simulink library "Mako_Lib"  (R2024b)
settings: Solver=VariableStepAuto  StartTime=0.0  StopTime=10.0  RelTol=1e-3
settings Model: Creator=pinto  LastModifiedBy=pinto

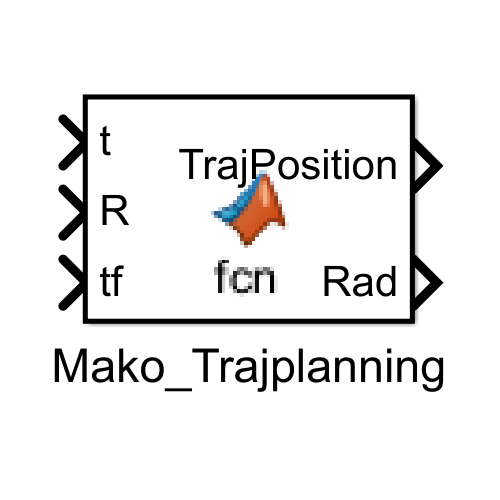
[thumbnail: Simulink's stored preview of the top-level diagram]
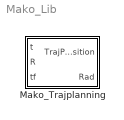
== system Mako_Lib ==
  Mako_Trajplanning : MATLAB Function  TreatAsAtomicUnit=on

== matlab function Mako_Lib/Mako_Trajplanning ==
  data: t input; TrajPosition output; R input; tf input; Rad output
function [TrajPosition,Rad] = Mako_Trajplanning(t,R,tf)
%#codegen

%    This function was generated by the Symbolic Math Toolbox version 24.2.
%    11-Jun-2025 20:14:08

% t = complex(t);  % if required to enforce complex operations
% R = complex(R);  % if required to enforce complex operations
% tf = complex(tf);  % if required to enforce complex operations
t2 = t.^2;
t3 = t.^3;
t4 = tf.^3;
t5 = 1.0./R;
t6 = 1.0./tf.^2;
t9 = sqrt(2.0);
t10 = pi.*(3.0./4.0);
t23 = R.*6.71238898038469;
t7 = 1.0./t4;
t8 = t3.*2.0;
t11 = t2.*tf.*3.0;
t13 = t9./2.0;
t17 = t4.*5.62949953421312e+14;
t18 = t4.*3.215789110431977e+15;
t19 = t3.*7.557478127706578e+15;
t21 = t2.*tf.*1.133621719155987e+16;
t26 = R.*t2.*t6.*2.013716694115407e+1;
t12 = -t11;
t14 = -t13;
t22 = -t21;
t24 = R.*t3.*t7.*1.342477796076938e+1;
t27 = -t26;
t15 = t4+t8+t12;
t25 = -t24;
t28 = t17+t19+t22;
t29 = t18+t19+t22;
t35 = R+t24+t27;
t41 = t23+t24+t27;
t34 = t25+t26;
if ~all(cellfun(@isscalar,{R,t15,t28,t29,tf}))
    error(message('symbolic:sym:matlabFunction:ConditionsMustBeScalar'));
end
if (0.0 <= R.*t28.*tf)
    t0 = t13.*t34;
elseif (0.0 <= R.*t29.*tf)
    t0 = R.*t9+R.*cos(t10+t5.*t35);
elseif (0.0 <= R.*t15.*tf)
    t0 = t13.*t41;
else
    t0 = NaN;
end
if ~all(cellfun(@isscalar,{R,t15,t28,t29,tf}))
    error(message('symbolic:sym:matlabFunction:ConditionsMustBeScalar'));
end
if (0.0 <= R.*t28.*tf)
    t1 = t9.*t34.*(-1.0./2.0);
elseif (0.0 <= R.*t29.*tf)
    t1 = -R.*sin(t10+t5.*t35);
elseif (0.0 <= R.*t15.*tf)
    t1 = t13.*t41;
else
    t1 = NaN;
end
TrajPosition = [t0;t1;1.0./5.0];
if nargout > 1
    if ~all(cellfun(@isscalar,{R,t15,t28,t29,tf}))    error(message('symbolic:sym:matlabFunction:ConditionsMustBeScalar'));end;if (0.0 <= R.*t28.*tf)    t0 = t13;elseif (0.0 <= R.*t29.*tf)    t0 = -cos(t10+t5.*t35);elseif (0.0 <= R.*t15.*tf)    t0 = t13;else    t0 = NaN;end;if ~all(cellfun(@isscalar,{R,t15,t28,t29,tf}))    error(message('symbolic:sym:matlabFunction:ConditionsMustBeScalar'));end;if (0.0 <= R.*t28.*tf)    t1 = t13;elseif (0.0 <= R.*t29.*tf)    t1 = sin(t10+t5.*t35);elseif (0.0 <= R.*t15.*tf)    t1 = t14;else    t1 = NaN;end;if ~all(cellfun(@isscalar,{R,t15,t28,t29,tf}))    error(message('symbolic:sym:matlabFunction:ConditionsMustBeScalar'));end;if (0.0 <= R.*t28.*tf)    t2 = t13;elseif (0.0 <= R.*t29.*tf)    t2 = sin(t10+t5.*t35);elseif (0.0 <= R.*t15.*tf)    t2 = t14;else    t2 = NaN;end;if ~all(cellfun(@isscalar,{R,t15,t28,t29,tf}))    error(message('symbolic:sym:matlabFunction:ConditionsMustBeScalar'));end;if (0.0 <= R.*t28.*tf)    t3 = t14;elseif (0.0 <= R.*t29.*tf)    t3 = cos(t10+t5.*t35);elseif (0.0 <= R.*t15.*tf)    t3 = t14;else    t3 = NaN;end;Rad = reshape([0.0,0.0,-1.0,t0,t1,0.0,t2,t3,0.0],[3,3]);
end
end
